simulink model "BME_project_Robust"  (R2020a)
settings: Solver=VariableStepAuto  StartTime=0.0  StopTime=100  RelTol=1e-3
settings Model: Creator=sunda  LastModifiedBy=sunda

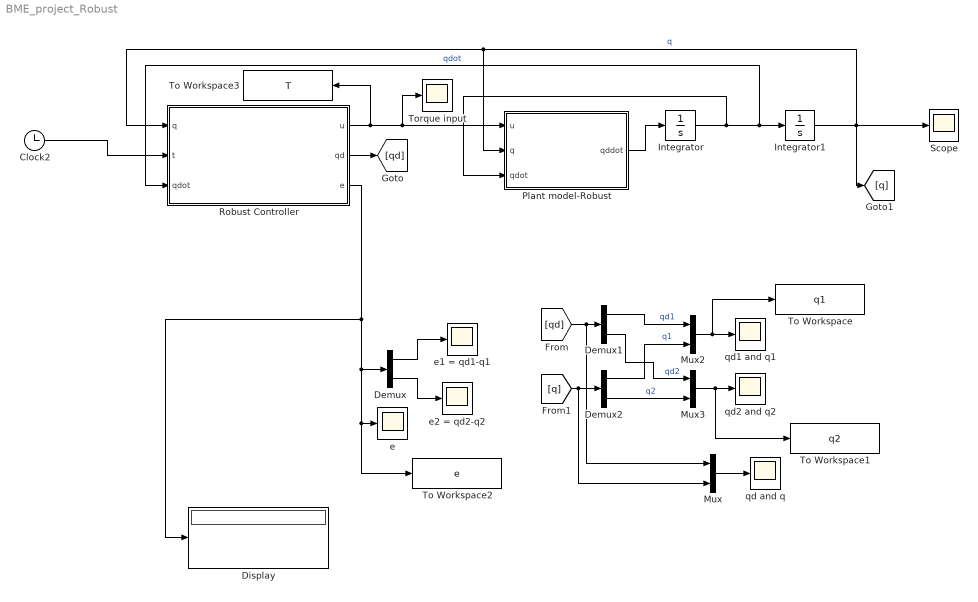
== system BME_project_Robust ==
  Clock2 : Clock
  Demux : Demux  Outputs=2
  Demux1 : Demux  Outputs=2
  Demux2 : Demux  Outputs=2
  Display : Display
  Integrator : Integrator  InitialCondition=zeros(2,1)
  Integrator1 : Integrator  InitialCondition=zeros(2,1)
  Mux : Mux  Inputs=2
  Mux2 : Mux  Inputs=2
  Mux3 : Mux  Inputs=2
  Plant model-Robust : MATLAB Function  TreatAsAtomicUnit=on
  Robust Controller : MATLAB Function  TreatAsAtomicUnit=on
  Scope : Scope
  To Workspace : ToWorkspace  VariableName=q1  SaveFormat=Timeseries  SampleTime=-1
  To Workspace1 : ToWorkspace  VariableName=q2  SaveFormat=Timeseries  SampleTime=-1
  To Workspace2 : ToWorkspace  VariableName=e  SaveFormat=Timeseries  SampleTime=-1
  To Workspace3 : ToWorkspace  VariableName=T  SaveFormat=Timeseries  SampleTime=-1
  Torque input : Scope
  e : Scope
  e1 = qd1-q1 : Scope
  e2 = qd2-q2 : Scope
  qd and q : Scope
  qd1 and q1 : Scope
  qd2 and q2 : Scope
  wires:
  Clock2/1 -> Robust Controller/2(t)
  Integrator/1 -> Plant model-Robust/3(qdot), Integrator1/1, Robust Controller/3(qdot)  "qdot"
  Integrator1/1 -> Plant model-Robust/2(q), Robust Controller/1(q), Scope/1, [q]  "q"
  Plant model-Robust/1(qddot) -> Integrator/1
  Robust Controller/1(u) -> To Workspace3/1, Torque input/1, Plant model-Robust/1(u)
  Demux2/2 -> Mux3/2  "q2"
  Demux1/2 -> Mux3/1  "qd2"
  Demux2/1 -> Mux2/2  "q1"
  Demux1/1 -> Mux2/1  "qd1"
  Mux3/1 -> To Workspace1/1, qd2 and q2/1
  [qd] -> Mux/1, Demux1/1
  Mux/1 -> qd and q/1
  Demux/2 -> e2 = qd2-q2/1
  [q] -> Mux/2, Demux2/1
  Robust Controller/3(e) -> Display/1, Demux/1, To Workspace2/1, e/1
  Demux/1 -> e1 = qd1-q1/1
  Robust Controller/2(qd) -> [qd]
  Mux2/1 -> To Workspace/1, qd1 and q1/1

== matlab function BME_project_Robust/Robust Controller ==
  data: q input; u output; t input; qdot input; qd output; e output
%% Robust controller

function [u,qd,e] = fcn(q,t,qdot)

q1 = q(1);
q2 = q(2);

q1dot =qdot(1);
q2dot = qdot(2);

  
qd = [cos(t) cos(2*t)]';
qd_dot = [-sin(t) -2*sin(2*t)]';
qd_ddot = [-cos(t) -4*cos(2*t)]';

e = qd-q;
e_dot =qd_dot - qdot;


% Gain values

alpha = 1.8; 
K = 42*eye(2);

r = e_dot + alpha *e;
 
Y = [qd_ddot(1)+alpha*e_dot(1)   qd_ddot(2)+alpha*e_dot(2)      2*cos(q2)*(qd_ddot(1)+alpha*e_dot(1))+cos(q2)*qd_ddot(2)+alpha*e_dot(2)-sin(q2)*q2dot*(qd_dot(1)+alpha*e(1))-sin(q2)*(q1dot+q2dot)*(qd_dot(2)+alpha*e(2))   q1dot   0;...
            0          qd_ddot(1)+alpha*e_dot(1)+qd_ddot(2)+alpha*e_dot(2)      cos(q2)*(qd_ddot(1)+alpha*e_dot(1))+sin(q2)*q1dot*(qd_dot(1)+alpha*e(1))    0   q2dot];

%%% Rho should upper bound Y*theta
Qddot_approx = [3;3];
Qdot_approx = [3;3];
M_approx = [5 0.5;0.5 0.5];
Vm_approx = [-1.5    -2; 1 0.5];
fd_approx = [6 0;0.5 2];
Rho=M_approx*Qddot_approx+Vm_approx*Qdot_approx+fd_approx*Qdot_approx;% +alpha*M_approx*[2; 2];
Rho;
% Rho = [20 20];

%%% Control law - Adaptive

u = Rho'*sign(r) +K*r;

end

== matlab function BME_project_Robust/Plant model-Robust ==
  data: u input; q input; qdot input; qddot output
%% Robot Plant model - Robust
function qddot = fcn(u,q,qdot)

q1 = q(1);
q2 = q(2);

q1dot =qdot(1);
q2dot = qdot(2);

p1 = 3.473; %%% kg.m^2
p2 = 0.196; %%% kg.m^2
p3 = 0.242; %%% kg.m^2

fd1 = 5.3; %%% N.m.sec
fd2 = 1.1; %%% N.m.sec
%%% Disturbance
% Td1 = 0.35;   %%% N.m
% Td2 = 0.35;   %%% N.m
% %% No disturbance
Td1 = 0;   %%% N.m
Td2 = 0;   %%% N.m
%%% Inertia matrix M(q)
M =[p1+2*p3*cos(q2)     p2 + p3*cos(q2);...
    p2 + p3* cos(q2)        p2];

%%% Centripetal and Coriollis term V(q,qdot)

Vm = [-p3*sin(q2)*q2dot     -p3*sin(q2)*(q1dot +q2dot);...
     p3* sin(q2)*q1dot                  0];
 
%%% Damping/ friction term 

Fd = [fd1   0;
      0     fd2];
  
%%% Disturbance:

Td = [Td1 Td2]';
%%% Robot dynamics of a Two - link Robot

qddot = inv(M)*(u - Vm*qdot -Fd*qdot - Td);

end
